simulink model "rtwdemo_lct_cpp"  (Simulink 7.6)
settings: Solver=FixedStepDiscrete  StartTime=0.0  StopTime=10  FixedStep=0.1  RelTol=1e-3
libraries: rtwdemowidgets x1
Description:
  | C++ Object Methods
settings Model: Creator=The MathWorks Inc.  ExtModeAutoUpdateStatusClock=off
settings MATStruct: SampleTime=0.1  Offset=0  Priority=[20.0]
settings DataIOCC: SaveOutput=off  SaveTime=off  SignalLoggingName=logsOut
settings OptimizationCC: InlineParams=on  InlineInvariantSignals=on  ZeroExternalMemoryAtStartup=off  ZeroInternalMemoryAtStartup=off  NoFixptDivByZeroProtection=on  EfficientFloat2IntCast=on  OptimizeModelRefInitCode=on  LifeSpan=1
settings DebuggingCC: SolverPrmCheckMsg=none  StrictBusMsg=ErrorOnBusTreatedAsVector
settings HardwareCC: ProdIntDivRoundTo=Zero  ProdEndianess=LittleEndian  ProdHWDeviceType=Generic->32-bit Embedded Processor  TargetHWDeviceType=Generic->32-bit Embedded Processor
settings ModelReferenceCC: ModelReferenceNumInstancesAllowed=Zero
settings RTWCC: SystemTargetFile=ert.tlc  TLCOptions=-aIncludeERTFirstTime=0  TemplateMakefile=ert_default_tmf  Description=Real-Time Workshop Embedded Coder (no auto configuration)  GenerateReport=on  RTWVerbose=off  ProcessScript=ert_make_rtw_hook  IncludeHyperlinkInReport=on  LaunchReport=on  TargetLang=C++
settings CodeAppCC: IgnoreCustomStorageClasses=off
settings ERTTargetCC: TargetFcnLib=ansi_tfl_tmw.mat  MultiwordLength=2048  GenerateSampleERTMain=on  SupportNonFinite=off  InlinedParameterPlacement=NonHierarchical  ERTCustomFileTemplate=example_file_process.tlc  ConvertIfToSwitch=off

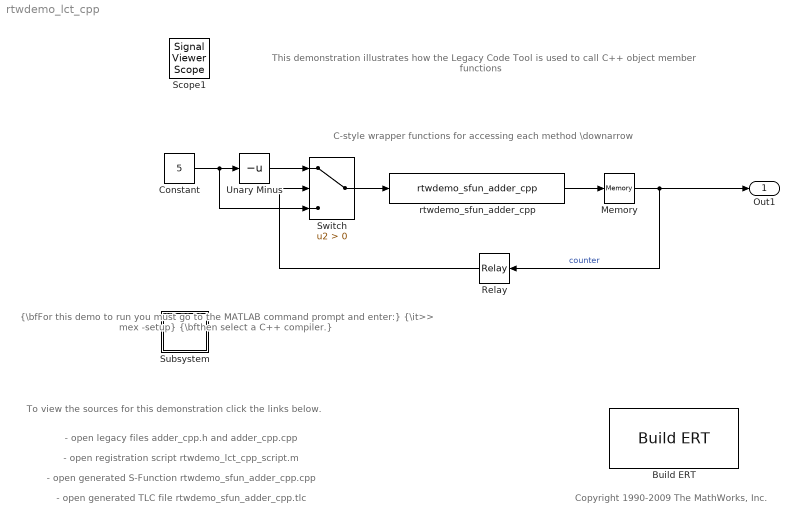
== system rtwdemo_lct_cpp ==
  note: C-style wrapper functions
      | for accessing each method
      | \downarrow
  note: {\bfFor this demo to run you must go to the MATLAB command prompt and enter:} {\it>> mex -setup}
      | {\bfthen select a C++ compiler.}
  note: This demonstration illustrates how the Legacy Code Tool is used to
      | call C++ object member functions
  note: Copyright 1990-2009 The MathWorks, Inc.
  note: - open legacy files adder_cpp.h and adder_cpp.cpp
  note: To view the sources for this demonstration
      | click the links below.
  note: - open registration script rtwdemo_lct_cpp_script.m
  note: - open generated S-Function rtwdemo_sfun_adder_cpp.cpp
  note: - open generated TLC file rtwdemo_sfun_adder_cpp.tlc
  Build ERT : rtwdemowidgets/Build ERT  SystemSampleTime=-1  attrib_overrides={'IncludeMdlTerminateFcn'}
  Constant : Constant  Value=5  OutDataTypeStr=int32
  Memory : Memory  InheritSampleTime=on  StateIdentifier=memCounter
      settings: RTWStateStorageClass=ExportedGlobal
  Relay : Relay  OnSwitchValue=101  OffSwitchValue=-1
  Subsystem : Subsystem
      mask init:
      | pos    = get_param(gcb, 'Position');
      | width  = pos(3) - pos(1);
      | height = pos(4) - pos(2);
      | 
      | marginPercent = 20;
      | marginPixels  = round(marginPercent / 100 * width);
      | 
      | x1 = width - marginPixels;
      | y1 = height;
      | x2 = width;
      | y2 = height - marginPixels;
      | x3 = width;
      | y3 = marginPixels;
      | x4 = width - marginPixels;
      | y4 = 0;
      | x5 = marginPixels;
      | y5 = 0;
      | x6 = 0;
      | y6 = marginPixels;
      | x7 = 0;
      | y7 = height - marginPixels;
      | x8 = marginPixels;
      | y8 = height;
      | 
      | xvec = [x1, x2, x3, x4, x5, x6, x7, x8];
      | yvec = [y1, y2, y3, y4, y5, y6, y7, y8];
      mask Display:
      | color('red');
      | patch(xvec, yvec);
      | color('white');
      | disp('!');
  Switch : Switch  Criteria=u2 > Threshold  ZeroCross=off
  Unary Minus : UnaryMinus
  rtwdemo_sfun_adder_cpp : S-Function  FunctionName=rtwdemo_sfun_adder_cpp  EnableBusSupport=off  mask(Legacy Function){SFunctionSpec=int32 y1 = adderOutput(int32 u1), ShowSpec=on}
      mask prompts: ShowSpec "Display function specification"
      mask help:
      | This block allows you to call the legacy functions specified by the following Legacy Code Tool definition:
      | def.SFunctionName = 'rtwdemo_sfun_adder_cpp';
      | def.OutputFcnSpec = 'int32 y1 = adderOutput(int32 u1)';
      | def.StartFcnSpec = 'createAdder()';
      | def.TerminateFcnSpec = 'deleteAdder()';
      | def.HeaderFiles = {'adder_cpp.h'};
      | def.SourceFiles = {'adder_cpp.cpp'};
      | def.IncPaths = {'sldemo_lct_src'};
      | def.SrcPaths = {'sldemo_lct_src'};
      | def.Options.useTlcWithAccel = false;
      | def.Options.language = 'C++';
      mask Help: <p>This block was generated automatically by the Legacy Code Tool. For detailed help on this tool, call<a href="matlab:legacy_code('help')"> legacy_code('help')</a>.</p>
      mask CallbackString:
      | |if strcmp(get_param(gcbh, 'ShowSpec'), 'on')
      |   set_param(gcbh, 'MaskDisplay', sprintf('fprintf(''%s'');', get_param(gcbh, 'SFunctionSpec')));
      | else
      |   set_param(gcbh, 'MaskDisplay', sprintf('fprintf(''%s'');', get_param(gcbh, 'FunctionName')));
      | end
      mask Display: fprintf('%s','int32 y1 = adderOutput(int32 u1)');
  Out1 : Outport
  Scope1 : SignalViewerScope  IOType=viewer  RefreshTime=0.035000
      settings: YMin=-20  YMax=120
  wires:
  Constant/1 -> Unary Minus/1, Switch/3
  Switch/1 -> rtwdemo_sfun_adder_cpp/1
  rtwdemo_sfun_adder_cpp/1 -> Memory/1
  Unary Minus/1 -> Switch/1
  Relay/1 -> Switch/2
  Memory/1 -> Relay/1, Out1/1  "counter"

== system rtwdemo_lct_cpp/Subsystem ==
